simulink model "DisturbanceTorques"  (R2023a)
settings: Solver=VariableStepAuto  StartTime=0.0  StopTime=tspan  RelTol=1e-3
values from neighbouring files (symbols this model uses):
  k = k+1    (= 1)    [A421_FinalProj_MainScript.m]    (also in WheelSizing_Script.m)
  mu = 398600    [A421_FinalProj_MainScript.m]    (also in WheelSizing_Script.m = 132712400000)
  rv_initial = [r_ECI;v_ECI]    [A421_FinalProj_MainScript.m]    (also in WheelSizing_Script.m)
undefined symbols (not defined in the file or in its folder): J, normal
settings Model: Creator=jself  LastModifiedBy=willb
settings DebuggingCC: UnconnectedInputMsg=warning  UnconnectedOutputMsg=warning  UnconnectedLineMsg=warning
settings ModelReferenceCC: EnableRefExpFcnMdlSchedulingChecks=on
settings RTWCC: DLArmComputeVersion=19.05

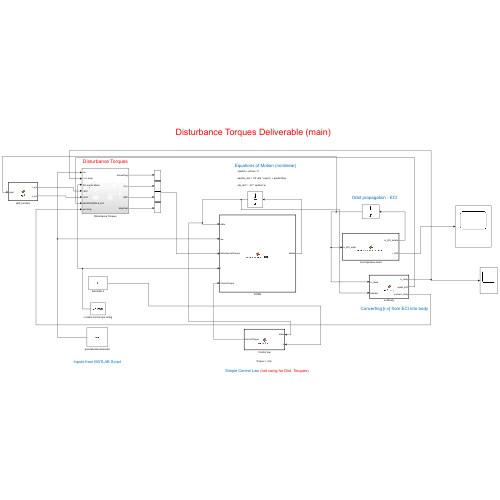
[thumbnail: Simulink's stored preview of the top-level diagram]
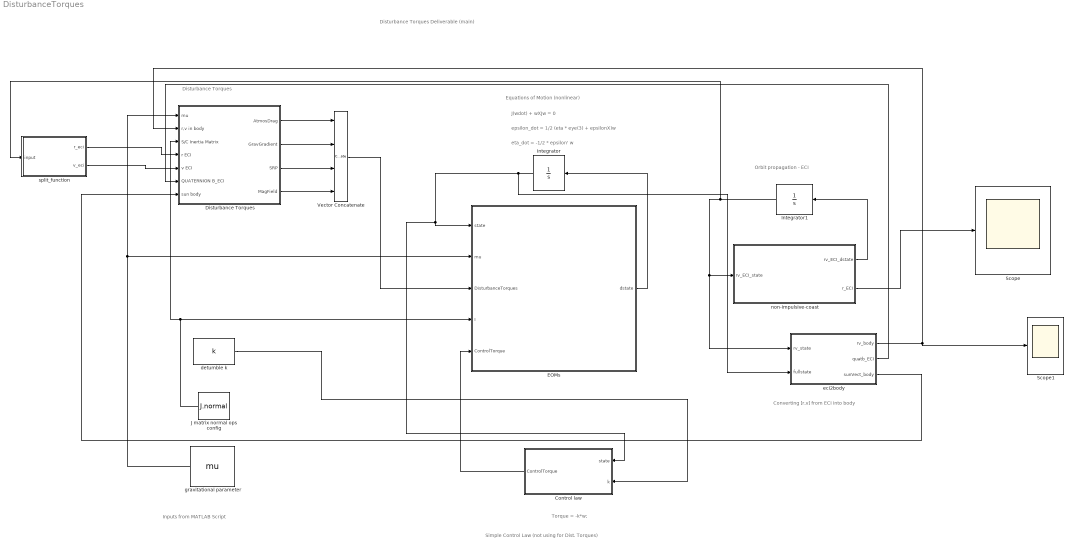
== system DisturbanceTorques ==
  note: Converting [r,v] from ECI into body
  note: Simple Control Law (not using for Dist. Torques)
  note: Torque = -k*w;
  note: eta_dot = -1/2 * epsilon' w
  note: epsilon_dot = 1/2 (eta * eye(3) + epsilonX)w
  note: J(wdot) + wXJw = 0
  note: Equations of Motion (nonlinear)
  note: Inputs from MATLAB Script
  note: Disturbance Torques Deliverable (main)
  note: Disturbance Torques
  note: Orbit propagation - ECI
  Control law : MATLAB Function  TreatAsAtomicUnit=on
  Disturbance Torques : Subsystem
  EOMs : MATLAB Function  TreatAsAtomicUnit=on
  Integrator : Integrator  InitialCondition=normal.state
  Integrator1 : Integrator  InitialCondition=rv_initial
  J matrix normal ops config : Constant  Value=J.normal
  Scope : Scope
  Scope1 : Scope
  Vector Concatenate : Concatenate  NumInputs=4
  detumble k : Constant  Value=k
  eci2body : MATLAB Function  TreatAsAtomicUnit=on
  gravitational parameter : Constant  Value=mu
  non-impulsive-coast : MATLAB Function  TreatAsAtomicUnit=on
  split_function : MATLAB Function  TreatAsAtomicUnit=on
  wires:
  EOMs/1(dstate) -> Integrator/1
  Integrator/1 -> eci2body/2(fullstate), Control law/1(state), EOMs/1(state)
  J matrix normal ops config/1 -> Disturbance Torques/3(S/C Inertia Matrix), EOMs/4(I)
  detumble k/1 -> Control law/2(k)
  Control law/1(ControlTorque) -> EOMs/5(ControlTorque)
  gravitational parameter/1 -> Disturbance Torques/1(mu), EOMs/2(mu)
  Disturbance Torques/1(AtmosDrag) -> Vector Concatenate/1
  Disturbance Torques/2(GravGradient) -> Vector Concatenate/2
  Disturbance Torques/3(SRP) -> Vector Concatenate/3
  Disturbance Torques/4(MagField) -> Vector Concatenate/4
  non-impulsive-coast/1(rv_ECI_dstate) -> Integrator1/1
  Integrator1/1 -> split_function/1(input), non-impulsive-coast/1(rv_ECI_state), eci2body/1(rv_state)
  non-impulsive-coast/2(r_ECI) -> Scope/1
  eci2body/1(rv_body) -> Scope1/1, Disturbance Torques/2(r,v in body)
  split_function/1(r_eci) -> Disturbance Torques/4(r ECI)
  split_function/2(v_eci) -> Disturbance Torques/5(v ECI)
  Vector Concatenate/1 -> EOMs/3(DisturbanceTorques)
  eci2body/2(quatb_ECI) -> Disturbance Torques/6(QUATERNION B_ECI)
  eci2body/3(sunVect_body) -> Disturbance Torques/7(sun body)

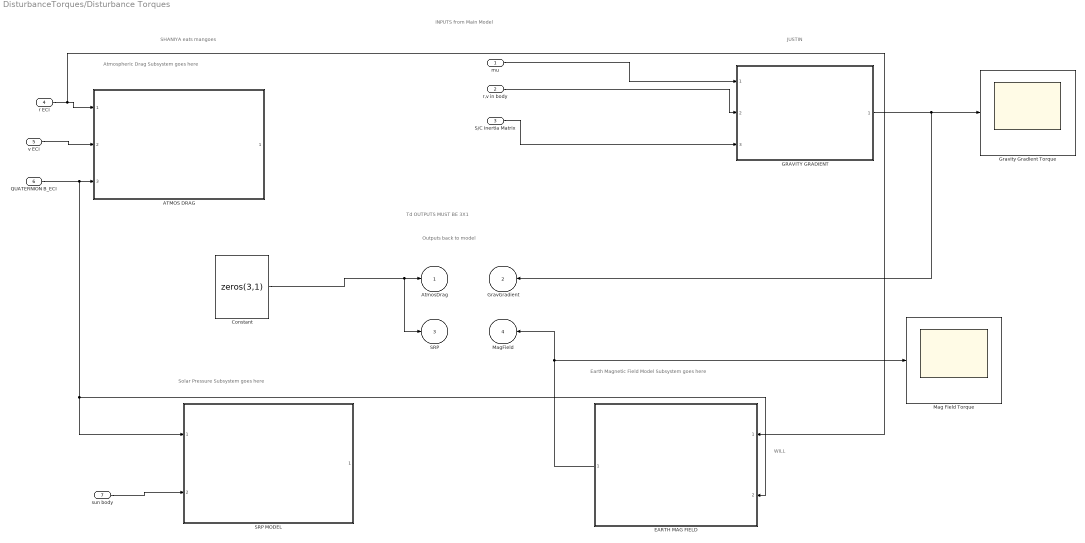
== system DisturbanceTorques/Disturbance Torques ==
  note: Solar Pressure Subsystem goes here
  note: INPUTS from Main Model
  note: WILL
  note: Earth Magnetic Field Model Subsystem goes here
  note: SHANIYA eats mangoes
  note: JUSTIN
  note: Atmospheric Drag Subsystem goes here
  note: Outputs back to model
  note: Td OUTPUTS MUST BE 3X1
  mu : Inport
  r,v in body : Inport  Port=2
  S/C Inertia Matrix : Inport  Port=3
  r ECI : Inport  Port=4
  v ECI : Inport  Port=5
  QUATERNION B_ECI : Inport  Port=6
  sun body : Inport  Port=7
  ATMOS DRAG : Subsystem  ReferencedSubsystem=AtmosphericDrag_SS
  Constant : Constant  Value=zeros(3,1)
  EARTH MAG FIELD : Subsystem  ReferencedSubsystem=EarthMagneticField_SS
  GRAVITY GRADIENT : Subsystem  ReferencedSubsystem=GravityGradient_SS
  Gravity Gradient Torque : Scope
  Mag Field Torque : Scope
  SRP MODEL : Subsystem  ReferencedSubsystem=SolarPressure_SS
  AtmosDrag : Outport
  GravGradient : Outport  Port=2
  SRP : Outport  Port=3
  MagField : Outport  Port=4
  wires:
  GRAVITY GRADIENT/1 -> GravGradient/1, Gravity Gradient Torque/1
  mu/1 -> GRAVITY GRADIENT/1
  r,v in body/1 -> GRAVITY GRADIENT/2
  S/C Inertia Matrix/1 -> GRAVITY GRADIENT/3
  r ECI/1 -> EARTH MAG FIELD/1, ATMOS DRAG/1
  v ECI/1 -> ATMOS DRAG/2
  EARTH MAG FIELD/1 -> MagField/1, Mag Field Torque/1
  Constant/1 -> SRP/1, AtmosDrag/1
  QUATERNION B_ECI/1 -> EARTH MAG FIELD/2, SRP MODEL/1, ATMOS DRAG/3
  sun body/1 -> SRP MODEL/2

== matlab function DisturbanceTorques/Control law ==
  data: state input; k input; ControlTorque output
function ControlTorque = controlLaw(state,k)

w = [state(1); state(2); state(3)];
ControlTorque = -k*w;

ControlTorque = ControlTorque .* 0;

end

== matlab function DisturbanceTorques/EOMs ==
  data: state input; mu input; DisturbanceTorques input; dstate output; I input; ControlTorque input
function dstate    = angularvelocity_ODE(state,mu,DisturbanceTorques,I,ControlTorque)

%{
This function is created for use in MATLAB's ode45 solver to compute the
following: 
    i.      Euler angle changes with time
    ii.     Quaternion changes with time
    iii.    Omega dot (change in angular velocity w.r.t time

INPUTS: 
    time = timespan for ode45
    state = mega state vector that contains all pertinent initial
    conditions. I.E., [omega; eulerangles, quaternion] 

state(1) = wx in body
state(2) = wy
state(3) = wz
state(4) = phi
state(5) = theta
state(6) = psi
state(7) = epsilonx in ECI
state(8) = epsilony
state(9) = epsilonz
state(10) = eta

I = inertia matrix (3x3) for the rigid body under consideration
T = net external torque (col vect) for system


OUTPUTS: derivative of the state for ode45 computation.
%}

%% Omega Dot

w = [state(1);
     state(2);
     state(3)];

% Find omega cross matrix
w_cross =   [   0      -w(3)     w(2);
                w(3)    0        -w(1);
               -w(2)    w(1)      0   ];


% Extract Td values
atmosTd = DisturbanceTorques(1:3);
gravTd = DisturbanceTorques(4:6);
srpTd = DisturbanceTorques(7:9);
magTd = DisturbanceTorques(10:12);

T = atmosTd + gravTd + srpTd + magTd + ControlTorque;

% Omega dot Equation of Motion
wdot = inv(I) * (T - w_cross * I * w);

%% Euler Angles

phi = state(4);
theta = state(5);
psi = state(6);

eulerdot = cos(theta)^(-1) * [   cos(theta)      sin(phi)*sin(theta)     cos(phi)*sin(theta); 
                                0               cos(phi)*cos(theta)     -sin(phi)*cos(theta);
                                0               sin(phi)                 cos(phi)           ] * w;

%% Quaternion Parameterization

epx = state(7);
epy = state(8);
epz = state(9);
eta = state(10);

epsilon = [epx; epy; epz];

epsilon_cross = [   0       -epz     epy;
                    epz     0        -epx;
                    -epy    epx      0    ];

% Derivatives of epsilon and eta
depsilon = 0.5 * (eta*eye(3) + epsilon_cross) * w;
deta = -0.5 * epsilon' * w;
quat = [depsilon(1); depsilon(2); depsilon(3); deta];

% Compile final output
dstate = [wdot;eulerdot;quat];                  % 10x1 coming out

end

== matlab function DisturbanceTorques/non-impulsive-coast ==
  data: rv_ECI_state input; rv_ECI_dstate output; r_ECI output
function [rv_ECI_dstate, r_ECI]  = non_impulsive_COAST(rv_ECI_state)
%{ 

*FOR COAST PHASE ONLY*

**This function assumes that thrust is exactly parallel to initial velocity
direction.

This function is for numerical integration (i.e., plug into ode45).
NOTE: only use this function for the BURN PHASE of the non-impulsive
maneuver. For the BURN phase, use "non_impulsive_BURN"

INPUTS: 
    INITIAL CONDITIONS
    state vector(1:3) = position (rx,ry,rz)
    state vector(4:6) = velocity (vx,vy,vz)

OUTPUT: New state vector after integration.
%%%%%%%%%%%%%%%%%%%%%%%%%%%%%%%%%%%%%%%%%%%%%%%%%
Justin Self, Cal Poly, Fall 2022; Introduction to Orbital Mechanics.
%%%%%%%%%%%%%%%%%%%%%%%%%%%%%%%%%%%%%%%%%%%%%%%%%
%}

mu = 398600; % km3/s2

rx = rv_ECI_state(1);
ry = rv_ECI_state(2);
rz = rv_ECI_state(3);
vx = rv_ECI_state(4);
vy = rv_ECI_state(5);
vz = rv_ECI_state(6);

r_vect = [rx ry rz];
r = norm(r_vect);

v_vect = [vx vy vz];
v = norm(v_vect);

xdot = vx;
ydot = vy;
zdot = vz;
xddot = (-mu*rx)/(r^3);
yddot = (-mu*ry)/(r^3);
zddot = (-mu*rz)/(r^3);

r_ECI = [xdot;ydot;zdot];

rv_ECI_dstate = [xdot; ydot; zdot; xddot; yddot; zddot];

end

== matlab function DisturbanceTorques/eci2body ==
  data: rv_state input; rv_body output; fullstate input; quatb_ECI output; sunVect_body output
function [rv_body,quatb_ECI,sunVect_body]  = eci2body(rv_state,fullstate)

sun_ECI = [1;0;0];

% Convert from ECI to body

r_eci = rv_state(1:3);
v_eci = rv_state(4:6);

epsilon_b_LVLH = fullstate(7:9);
eta_b_LVLH = fullstate(10);

[Cb_LVLH] = quat2rotationmatrix(epsilon_b_LVLH,eta_b_LVLH);                 % Find body - LVLH matrix

rmag_eci = norm(r_eci);                                                     % Find LVLH-ECI matrix
h_eci = cross(r_eci,v_eci);
hmag_eci = norm(h_eci);

% ECI to LVLH
z = -r_eci/rmag_eci;
y = -h_eci/hmag_eci;
x = cross(y,z);

C_LVLH_ECI = [x'; y'; z'];                                                  % From ECI to LVLH

% b to ECI rotation matrix
Cb_ECI = Cb_LVLH*C_LVLH_ECI;
C = Cb_ECI;                                                                 % easy 


% NEED QUATERNION RELATING BODY/ECI

% Matlab's way
q = rotm2quat(C); % eta, epsx, epsy, epsz
quatb_ECI = [q(2); q(3); q(4); q(1)]; % eps; eta

% FINALLY, convert r and v vectors from ECI into body
rv_body = [Cb_ECI * r_eci; Cb_ECI * v_eci];
sunVect_body = Cb_ECI * sun_ECI;

end

== matlab function DisturbanceTorques/split_function ==
  data: input input; r_eci output; v_eci output
function [r_eci,v_eci] = split(input)

r_eci = input(1:3);
v_eci = input(4:6);

end

% because I don't know a Simu funct that does this faster! -J
